simulink model "SimpleEngineSSCVDB"  (R2026b)
settings: Solver=VariableStepAuto
undefined symbols (not defined in the file): Afr, BSFC, CrkAng, EngSpdOut, EngTrq, ExhManGasTemp, FuelFlw, FuelVolFlw, IntkPortFlw, NormAirChrg
libraries: fl_lib x3, nesl_utility x2, simulink x2, autolibsharedcommon x1, autolibsharedmappedengines x1
settings Model: ModifiedByFormat=The MathWorks, Inc.  Creator=The MathWorks, Inc.  LastModifiedBy=The MathWorks, Inc.
settings OptimizationCC: ReuseModelBlockBuffer=off
settings RTWCC: DLArmComputeVersion=19.05

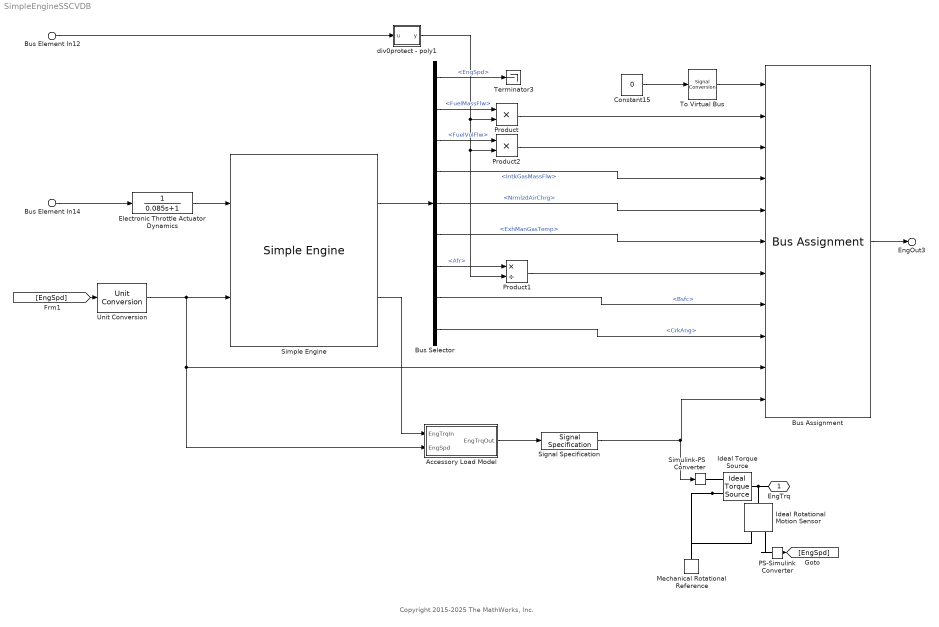
== system SimpleEngineSSCVDB ==
  note: Copyright 2015-2025 The MathWorks, Inc.
  Bus Element In12 : Inport  PortName=Cntrl  Element=Engine.ClsdLpFuelMult
  Bus Element In14 : Inport  PortName=Cntrl  Element=Engine.TrqCmd
  Accessory Load Model : Subsystem
  Bus Assignment : BusAssignment  AssignedSignals=FuelFlw,FuelVolFlw,IntkPortFlw,NormAirChrg,ExhManGasTemp,Afr,BSFC,CrkAng,EngSpdOut,EngTrq
  Bus Selector : BusSelector  OutputSignals=EngSpd,FuelMassFlw,FuelVolFlw,IntkGasMassFlw,NrmlzdAirChrg,ExhManGasTemp,Afr,Bsfc,CrkAng
  Constant15 : Constant  Value=0  OutDataTypeStr=Bus: EngineBUS  SampleTime=Inf
  Electronic Throttle Actuator Dynamics : TransferFcn  Denominator=[0.085 1]
  Ideal Rotational Motion Sensor : fl_lib/Mechanical/Mechanical Sensors/Ideal Rotational Motion Sensor  reference=foundation.enum.MeasurementReference.difference  acceleration_port=false  velocity_port=true  position_port=false  wrap_angle=false  offset=0 rad
  Ideal Torque Source : fl_lib/Mechanical/Mechanical Sources/Ideal Torque Source
  Mechanical Rotational Reference : fl_lib/Mechanical/Rotational Elements/Mechanical Rotational Reference
  PS-Simulink Converter : nesl_utility/PS-Simulink Converter  PhysicalDomain=network_engine_domain  SubClassName=ps_output  LeftPortType=input  RightPortType=output  PseudoPeriodic=off  Frequencies=[]  VectorFormat=inherit  Unit=rpm  AffineConversion=off
  Product : Product
  Product1 : Product  Inputs=*/
  Product2 : Product
  Signal Specification : SignalSpecification  Dimensions=1
  Simple Engine : autolibsharedmappedengines/Simple Engine  f_tqmax=[75.679776480773256 75.679776480773256 97.173658538143172 116.84042599160529 152.21029882684542 175 174.99889520597083 174.99996520122858 175 175 175 175 175 175 175 175]  f_tqmax_n_bpt=[0 750 1053.57142857143 1357.14285714286 1660.71428571429 1964.28571428571 2267.85714285714 2571.42857142857 2875 3178.57142857143 3482.14285714286 3785.71428571429 4089.28571428571 4392.85714285714 4696.42857142857 5000]  Lhv=46e6  Sg=0.745  BsfcAvg=350  aMode=2
      settings: LibrarySourceBlock=vdynlib/Powertrain/Propulsion/Simple Engine
  Simulink-PS Converter : nesl_utility/Simulink-PS Converter  PhysicalDomain=network_engine_domain  SubClassName=ps_input  LeftPortType=input  RightPortType=output  PseudoPeriodic=off  Frequencies=[]  NoiseDistribution=none  NoiseParameters=[]  Unit=N*m  AffineConversion=off  FilteringAndDerivatives=filter  SimscapeFilterOrder=2  InputFilterTimeConstant=0.01  UdotUserProvided=0
  Terminator3 : Terminator
  To Virtual Bus : SignalConversion  ConversionOutput=Virtual bus  OverrideOpt=off
  Unit Conversion : UnitConversion
  div0protect - poly1 : Subsystem  mask{thresh=0.01, ZeroCross=on, ZeroCross1=off}
      mask prompts: thresh "threshold"; ZeroCross "Simulink:blkprm_prompts:AllBlksEnableZC"
      mask TypeOptions ZeroCross: Switch/ZeroCross | Switch1/ZeroCross
      mask DialogControl ParamGroup Prompt: Threshold
      mask DialogControl ZeroCross Prompt: Enable zero-crossing detection
  EngTrq : PMIOPort  Side=Right
  EngOut3 : Outport  PortName=EngFdbk
  wires:
  Simple Engine/2 -> Accessory Load Model/1(EngTrqIn)
  Bus Selector/9 -> Bus Assignment/9  "<CrkAng>"
  Bus Selector/1 -> Terminator3/1  "<EngSpd>"
  Product/1 -> Bus Assignment/2
  Bus Selector/6 -> Bus Assignment/6  "<ExhManGasTemp>"
  Bus Element In12/1 -> div0protect - poly1/1(u)
  [EngSpd] -> Unit Conversion/1
  Accessory Load Model/1(EngTrqOut) -> Signal Specification/1
  Bus Selector/5 -> Bus Assignment/5  "<NrmlzdAirChrg>"
  div0protect - poly1/1(y) -> Product/2, Product1/2, Product2/2
  Bus Selector/3 -> Product2/1  "<FuelVolFlw>"
  Bus Element In14/1 -> Electronic Throttle Actuator Dynamics/1
  Product1/1 -> Bus Assignment/7
  Bus Selector/4 -> Bus Assignment/4  "<IntkGasMassFlw>"
  Bus Selector/7 -> Product1/1  "<Afr>"
  Bus Selector/2 -> Product/1  "<FuelMassFlw>"
  Electronic Throttle Actuator Dynamics/1 -> Simple Engine/1
  Product2/1 -> Bus Assignment/3
  Simple Engine/1 -> Bus Selector/1
  Bus Selector/8 -> Bus Assignment/8  "<Bsfc>"
  Unit Conversion/1 -> Accessory Load Model/2(EngSpd), Bus Assignment/10, Simple Engine/2
  To Virtual Bus/1 -> Bus Assignment/1
  Constant15/1 -> To Virtual Bus/1
  Bus Assignment/1 -> EngOut3/1
  PS-Simulink Converter/1 -> [EngSpd]
  Signal Specification/1 -> Simulink-PS Converter/1, Bus Assignment/11
  connections:
  Ideal Rotational Motion Sensor/LConn1 -- Ideal Torque Source/LConn1 -- EngTrq/RConn1
  Ideal Torque Source/RConn2 -- Ideal Rotational Motion Sensor/RConn1 -- Mechanical Rotational Reference/LConn1
  PS-Simulink Converter/LConn1 -- Ideal Rotational Motion Sensor/RConn2
  Simulink-PS Converter/RConn1 -- Ideal Torque Source/RConn1

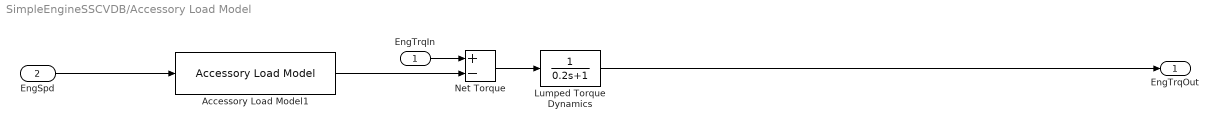
== system SimpleEngineSSCVDB/Accessory Load Model ==
  EngTrqIn : Inport
  EngSpd : Inport  Port=2
  Accessory Load Model1 : autolibsharedcommon/Accessory Load Model  AccPwrTbl=PlntEngAccPwrTbl  AccSpdBpts=PlntEngAccSpdBpt  aMode=aMode
  Lumped Torque Dynamics : TransferFcn  Denominator=[0.2 1]
  Net Torque : Sum  Inputs=+-
  EngTrqOut : Outport  Unit=N*m  VectorParamsAs1DForOutWhenUnconnected=off
  wires:
  Accessory Load Model1/1 -> Net Torque/2
  Lumped Torque Dynamics/1 -> EngTrqOut/1
  EngSpd/1 -> Accessory Load Model1/1
  Net Torque/1 -> Lumped Torque Dynamics/1
  EngTrqIn/1 -> Net Torque/1

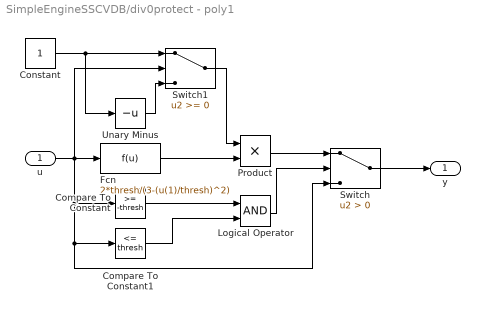
== system SimpleEngineSSCVDB/div0protect - poly1 ==
  u : Inport
  Compare To Constant : simulink/Logic and Bit Operations/Compare To Constant  relop=>=  const=-thresh  OutDataTypeStr=boolean  ZeroCross=off
  Compare To Constant1 : simulink/Logic and Bit Operations/Compare To Constant  relop=<=  const=thresh  OutDataTypeStr=boolean  ZeroCross=off
  Constant : Constant
  Fcn : Fcn  Expr=2*thresh/(3-(u(1)/thresh)^2)
  Logical Operator : Logic  AllPortsSameDT=off  OutDataTypeStr=boolean
  Product : Product
  Switch : Switch  Criteria=u2 > Threshold  SaturateOnIntegerOverflow=off  InputSameDT=off
  Switch1 : Switch  SaturateOnIntegerOverflow=off  InputSameDT=off
  Unary Minus : UnaryMinus
  y : Outport  VectorParamsAs1DForOutWhenUnconnected=off
  wires:
  u/1 -> Switch/3, Compare To Constant1/1, Compare To Constant/1, Switch1/2, Fcn/1
  Fcn/1 -> Product/2
  Logical Operator/1 -> Switch/2
  Compare To Constant/1 -> Logical Operator/1
  Compare To Constant1/1 -> Logical Operator/2
  Switch/1 -> y/1
  Switch1/1 -> Product/1
  Constant/1 -> Switch1/1, Unary Minus/1
  Unary Minus/1 -> Switch1/3
  Product/1 -> Switch/1
